simulink model "Deploy_Simulink_R2015b"  (R2015b)
settings: Solver=ode1  StartTime=0.0  StopTime=inf  FixedStep=0.004  RelTol=1e-3
values from neighbouring files (symbols this model uses):
  elev_0 = -27.5*pi/180    (= -0.479965544298)    [setup_lab_heli_3d.m]
  K_AMP = 3    [setup_lab_heli_3d.m]
  K_EC_E = - 2 * pi / ( 4 * 1024 )    (= -0.00153398078789)    [setup_heli_3d_configuration.m]
  K_EC_P = 2 * pi / ( 4 * 1024 )    (= 0.00153398078789)    [setup_heli_3d_configuration.m]
  K_EC_T = 2 * pi / ( 8 * 1024 )    (= 0.000766990393943)    [setup_heli_3d_configuration.m]
  lambdaSplit = reshape(lambda, lambdaDim,  sizeSeg,DoP)    [Simulink_Setup.m]
  LAMBDASplit = reshape(LAMBDA, xDim, xDim, sizeSeg,DoP)    [Simulink_Setup.m]
  pSplit = reshape(par,    pDim,       sizeSeg,DoP)    [Simulink_Setup.m]
  uSplit = reshape(u,      uDim,       sizeSeg,DoP)    [Simulink_Setup.m]
  VMAX_AMP = 24    [setup_lab_heli_3d.m]
  VMAX_DAC = 10    [setup_lab_heli_3d.m]
  wcf = 2 * pi * 4    (= 25.1327412287)    [setup_lab_heli_3d.m]
  xSplit = reshape(x,      xDim,       sizeSeg,DoP)    [Simulink_Setup.m]
  zetaf = 0.9    [setup_lab_heli_3d.m]
undefined symbols (not defined in the file or in its folder): HIL, qc_get_step_size
libraries: quarc_library x4
settings Model: SimulationMode=external  Creator=Deng  LastModifiedBy=deng
settings SolverCC: PositivePriorityOrder=on
settings DataIOCC: LimitDataPoints=off
settings OptimizationCC: SimCompilerOptimization=on
settings DebuggingCC: AllowSymbolicDim=on
settings HardwareCC: ProdBitPerPointer=32  ProdLargestAtomicFloat=None  ProdWordSize=32  ProdHWDeviceType=Custom Processor->Custom
settings ModelReferenceCC: PropagateSignalLabelsOutOfModel=on
settings SFSimCC: SimCustomHeaderCode="#include \"NMPC_Iter.h\""  SimUserSources=NMPC_Iter.c OCP_F_Fu_Fx.c  SimUserLibraries=NMPC_Iter.lib
settings SFSimCC: SimUserIncludeDirs=|
  | .\codegen\lib\NMPC_Iter
  | .\codegen\lib\OCP_F_Fu_Fx
settings RTWCC: SystemTargetFile=quarc_win64.tlc  TemplateMakefile=quarc_default_tmf  Description=QUARC Win64 Target  GenerateReport=on  RTWUseSimCustomCode=on  CustomHeaderCode="#include \"NMPC_Iter.h\""  CustomSource=NMPC_Iter.c OCP_F_Fu_Fx.c  CustomLibrary=NMPC_Iter.lib  BuildConfiguration=Faster Runs  LaunchReport=on
settings RTWCC: CustomInclude=|
  | .\codegen\lib\NMPC_Iter
  | .\codegen\lib\OCP_F_Fu_Fx
settings STFCustomTargetCC: GeneratePreprocessorConditionals=Use local settings  CPPClassGenCompliant=off
settings GRTTargetCC: ParMdlRefBuildCompliant=off  CompOptLevelCompliant=off  CombineOutputUpdateFcns=off  MatFileLogging=off  CPPClassGenCompliant=off  GRTInterface=on  UseToolchainInfoCompliant=off  ExtMode=on  ExtModeMexFile=quarc_comm

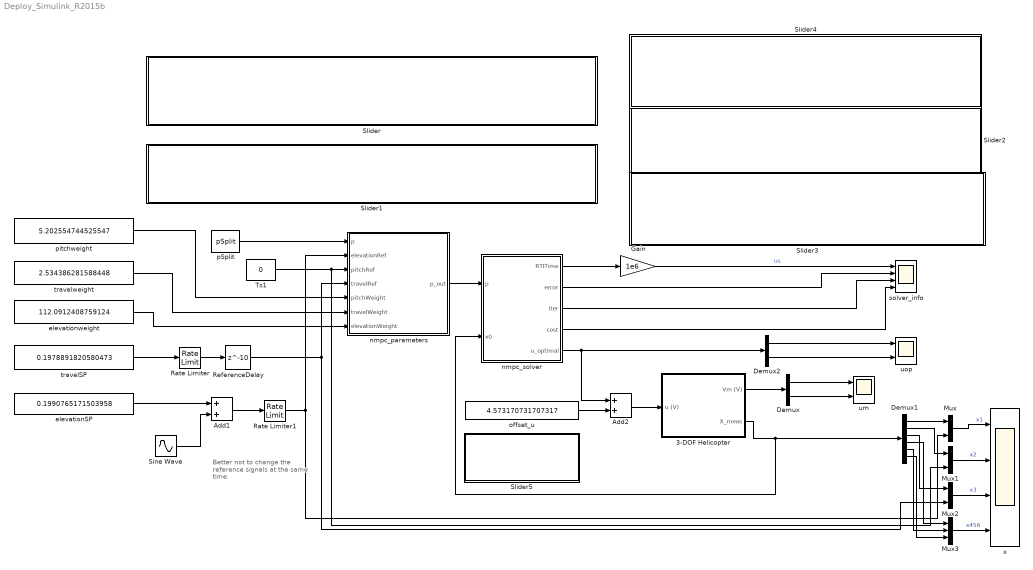
== system Deploy_Simulink_R2015b ==
  note: Better not to change the reference signals at the same time.
  3-DOF Helicopter : Subsystem
  Add1 : Sum
  Add2 : Sum
  Demux : Demux  Outputs=2
  Demux1 : Demux  Outputs=6
  Demux2 : Demux  Outputs=2
  Gain : Gain  Gain=1e6
  Mux : Mux  Inputs=2
  Mux1 : Mux  Inputs=2
  Mux2 : Mux  Inputs=2
  Mux3 : Mux  Inputs=3
  Rate Limiter : RateLimiter  RisingSlewLimit=2  FallingSlewLimit=-2  SampleTimeMode=inherited
  Rate Limiter1 : RateLimiter  RisingSlewLimit=50  FallingSlewLimit=-50  SampleTimeMode=inherited
  ReferenceDelay : Delay  DelayLength=10  InitialCondition=0
  Sine Wave : Sin  Amplitude=0  Frequency=0.5  SampleTime=0
  Slider : Subsystem  DialogController=hmiCreateDDGDialog  IsWebBlock=on  mask(MWDashboardBlock){webBlockId=958bdc94-fbbd-4d66-a7c2-c7b380b51c1f, webBlockType=slider, ShowInLibBrowser=on, ShowInitialText=on, HMISrcModelName=Simulink_C_Deploy_R2015b}
      mask prompts: webBlockId "WebBlock Id"; webBlockType "WebBlock Type"; HMISrcModelName "Source Model"
      mask Help: helpview([docroot '/mapfiles/simulink.map'], 'hmi_slider')
      mask Display:
      | if strcmp(get_param(bdroot(gcb),'BlockDiagramType'), 'library')
      |     image([(matlabroot) '/toolbox/simulink/hmi/icons/Slider.png']);
      | end
  Slider1 : Subsystem  DialogController=hmiCreateDDGDialog  IsWebBlock=on  mask(MWDashboardBlock){webBlockId=d0239637-77bd-428c-ab30-bd13650fc7b6, webBlockType=slider, ShowInLibBrowser=on, ShowInitialText=on, HMISrcModelName=Simulink_C_Deploy_R2015b}
      mask prompts: webBlockId "WebBlock Id"; webBlockType "WebBlock Type"; HMISrcModelName "Source Model"
      mask Help: helpview([docroot '/mapfiles/simulink.map'], 'hmi_slider')
      mask Display:
      | if strcmp(get_param(bdroot(gcb),'BlockDiagramType'), 'library')
      |     image([(matlabroot) '/toolbox/simulink/hmi/icons/Slider.png']);
      | end
  Slider2 : Subsystem  DialogController=hmiCreateDDGDialog  IsWebBlock=on  mask(MWDashboardBlock){webBlockId=9382aac3-409f-4dab-a4f9-baf18b7ce907, webBlockType=slider, ShowInLibBrowser=on, ShowInitialText=on, HMISrcModelName=Simulink_C_Deploy_R2015b}
      mask prompts: webBlockId "WebBlock Id"; webBlockType "WebBlock Type"; HMISrcModelName "Source Model"
      mask Help: helpview([docroot '/mapfiles/simulink.map'], 'hmi_slider')
      mask Display:
      | if strcmp(get_param(bdroot(gcb),'BlockDiagramType'), 'library')
      |     image([(matlabroot) '/toolbox/simulink/hmi/icons/Slider.png']);
      | end
  Slider3 : Subsystem  DialogController=hmiCreateDDGDialog  IsWebBlock=on  mask(MWDashboardBlock){webBlockId=d7a49558-d97e-4fdd-ae2b-0498040a2635, webBlockType=slider, ShowInLibBrowser=on, ShowInitialText=on, HMISrcModelName=Simulink_C_Deploy_R2015b}
      mask prompts: webBlockId "WebBlock Id"; webBlockType "WebBlock Type"; HMISrcModelName "Source Model"
      mask Help: helpview([docroot '/mapfiles/simulink.map'], 'hmi_slider')
      mask Display:
      | if strcmp(get_param(bdroot(gcb),'BlockDiagramType'), 'library')
      |     image([(matlabroot) '/toolbox/simulink/hmi/icons/Slider.png']);
      | end
  Slider4 : Subsystem  DialogController=hmiCreateDDGDialog  IsWebBlock=on  mask(MWDashboardBlock){webBlockId=5022bdd5-4ec7-4769-8c29-2847bff93344, webBlockType=slider, ShowInLibBrowser=on, ShowInitialText=on, HMISrcModelName=Simulink_C_Deploy_R2015b}
      mask prompts: webBlockId "WebBlock Id"; webBlockType "WebBlock Type"; HMISrcModelName "Source Model"
      mask Help: helpview([docroot '/mapfiles/simulink.map'], 'hmi_slider')
      mask Display:
      | if strcmp(get_param(bdroot(gcb),'BlockDiagramType'), 'library')
      |     image([(matlabroot) '/toolbox/simulink/hmi/icons/Slider.png']);
      | end
  Slider5 : Subsystem  DialogController=hmiCreateDDGDialog  IsWebBlock=on  mask(MWDashboardBlock){webBlockId=dba8a8ef-8cf2-4f6b-b7e7-21e88edd4f6f, webBlockType=slider, ShowInLibBrowser=on, ShowInitialText=on, HMISrcModelName=Simulink_C_Deploy_R2015b}
      mask prompts: webBlockId "WebBlock Id"; webBlockType "WebBlock Type"; HMISrcModelName "Source Model"
      mask Help: helpview([docroot '/mapfiles/simulink.map'], 'hmi_slider')
      mask Display:
      | if strcmp(get_param(bdroot(gcb),'BlockDiagramType'), 'library')
      |     image([(matlabroot) '/toolbox/simulink/hmi/icons/Slider.png']);
      | end
  Ts1 : Constant  Value=0
  elevationSP : Constant  Value=0.1990765171503958
  elevationweight : Constant  Value=112.0912408759124
  nmpc_parameters : MATLAB Function  TreatAsAtomicUnit=on
  nmpc_solver : Subsystem
  offset_u : Constant  Value=4.573170731707317
  pSplit : Constant  Value=pSplit
  pitchweight : Constant  Value=5.202554744525547
  solver_info : Scope  NumInputPorts=4
  travelSP : Constant  Value=0.1978891820580473
  travelweight : Constant  Value=2.534386281588448
  um : Scope  NumInputPorts=2
  uop : Scope  NumInputPorts=2
  x : Scope  NumInputPorts=4
  wires:
  pSplit/1 -> nmpc_parameters/1(p)
  nmpc_parameters/1(p_out) -> nmpc_solver/1(p)
  nmpc_solver/2(error) -> solver_info/2
  nmpc_solver/1(RTITime) -> Gain/1
  nmpc_solver/4(cost) -> solver_info/4
  nmpc_solver/3(iter) -> solver_info/3
  Gain/1 -> solver_info/1  "us"
  Ts1/1 -> nmpc_parameters/3(pitchRef), Mux1/2
  Demux/1 -> um/1
  Demux/2 -> um/2
  3-DOF Helicopter/2(X_meas) -> nmpc_solver/2(x0), Demux1/1
  Rate Limiter/1 -> ReferenceDelay/1
  Rate Limiter1/1 -> Mux/2, nmpc_parameters/2(elevationRef)
  Demux1/1 -> Mux/1
  Mux/1 -> x/1  "x1"
  Demux1/2 -> Mux1/1
  Mux1/1 -> x/2  "x2"
  Mux2/1 -> x/3  "x3"
  Demux1/3 -> Mux2/1
  Demux1/4 -> Mux3/1
  Demux1/5 -> Mux3/2
  Demux1/6 -> Mux3/3
  Mux3/1 -> x/4  "x456"
  ReferenceDelay/1 -> nmpc_parameters/4(travelRef), Mux2/2
  elevationSP/1 -> Add1/1
  Add1/1 -> Rate Limiter1/1
  Sine Wave/1 -> Add1/2
  travelSP/1 -> Rate Limiter/1
  Add2/1 -> 3-DOF Helicopter/1(u (V))
  3-DOF Helicopter/1(Vm (V)) -> Demux/1
  Demux2/1 -> uop/1
  Demux2/2 -> uop/2
  pitchweight/1 -> nmpc_parameters/5(pitchWeight)
  travelweight/1 -> nmpc_parameters/6(travelWeight)
  elevationweight/1 -> nmpc_parameters/7(elevationWeight)
  nmpc_solver/5(u_optimal) -> Add2/1, Demux2/1
  offset_u/1 -> Add2/2

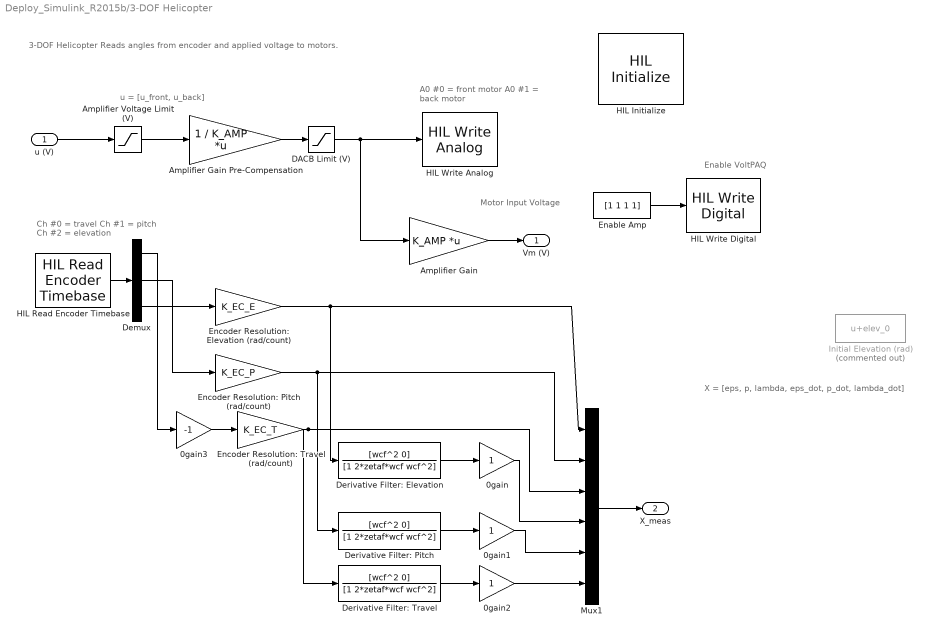
== system Deploy_Simulink_R2015b/3-DOF Helicopter ==
  note: A0 #0 = front motor
      | A0 #1 = back motor
  note: u = [u_front, u_back]
  note: Motor Input Voltage
  note: 3-DOF Helicopter
      | Reads angles from encoder and applied voltage to motors.
  note: Ch #0 = travel
      | Ch #1 = pitch
      | Ch #2 = elevation
  note: X = [eps, p, lambda, eps_dot, p_dot, lambda_dot]
  note: Enable VoltPAQ
  u (V) : Inport
  0gain : Gain
  0gain1 : Gain
  0gain2 : Gain
  0gain3 : Gain  Gain=-1
  Amplifier Gain : Gain  Gain=K_AMP  Multiplication=Matrix(K*u)  SaturateOnIntegerOverflow=on  OutDataTypeStr=Inherit: Same as input  ParamDataTypeStr=Inherit: Same as input
  Amplifier Gain Pre-Compensation : Gain  Gain=1 / K_AMP  Multiplication=Matrix(K*u)  SaturateOnIntegerOverflow=on  OutDataTypeStr=Inherit: Same as input  ParamDataTypeStr=Inherit: Same as input
  Amplifier Voltage Limit (V) : Saturate  UpperLimit=VMAX_AMP  LowerLimit=0
  DACB Limit (V) : Saturate  UpperLimit=VMAX_DAC  LowerLimit=-VMAX_DAC
  Demux : Demux  Outputs=3
  Derivative Filter: Elevation : TransferFcn  Numerator=[wcf^2 0]  Denominator=[1 2*zetaf*wcf wcf^2]
  Derivative Filter: Pitch : TransferFcn  Numerator=[wcf^2 0]  Denominator=[1 2*zetaf*wcf wcf^2]
  Derivative Filter: Travel : TransferFcn  Numerator=[wcf^2 0]  Denominator=[1 2*zetaf*wcf wcf^2]
  Enable Amp : Constant  Value=[1 1 1 1]
  Encoder Resolution: Elevation (rad/count) : Gain  Gain=K_EC_E
  Encoder Resolution: Pitch (rad/count) : Gain  Gain=K_EC_P
  Encoder Resolution: Travel (rad/count) : Gain  Gain=K_EC_T
  HIL Initialize : quarc_library/Data Acquisition/Generic/Configuration/HIL Initialize  object_name=HIL-1  board_type=q8_usb  board_number=0  board_options=update_rate=normal  exclusive=off  active=on  hardware_clocks=[0:2]  clock_modes=[]  initial_clock_frequencies=[]  set_clock_params_at_start=off  set_clock_params_at_switch_in=off  set_clock_frequencies_at_start=off  set_clock_frequencies_at_switch_in=off  analog_input_channels=[0:7]  analog_input_configurations=[]  analog_input_maximums=10  analog_input_minimums=-10  set_analog_input_params_at_start=on  set_analog_input_params_at_switch_in=off  analog_output_channels=[0:7]  analog_output_maximums=10  analog_output_minimums=-10  initial_analog_outputs=[0]  final_analog_outputs=[0]  watchdog_analog_outputs=0  set_analog_output_params_at_start=on  set_analog_output_params_at_switch_in=off  set_analog_outputs_at_start=on  set_analog_outputs_at_switch_in=off  set_analog_outputs_at_terminate=on  set_analog_outputs_at_switch_out=off  set_analog_outputs_on_watchdog=off  digital_input_channels=[4:7]  digital_output_channels=[0:3]  digital_output_configuration=[]  initial_digital_outputs=[0]  final_digital_outputs=[0]  watchdog_digital_outputs=[0]  set_digital_output_params_at_start=off  set_digital_output_params_at_switch_in=off  set_digital_outputs_at_start=on  set_digital_outputs_at_switch_in=off  set_digital_outputs_at_terminate=on  set_digital_outputs_at_switch_out=off  set_digital_outputs_on_watchdog=off  encoder_channels=[0:7]  quadrature=[4]  encoder_filter_frequency=[]  initial_encoder_counts=[0]  set_encoder_params_at_start=on  set_encoder_params_at_switch_in=off  set_encoder_counts_at_start=on  set_encoder_counts_at_switch_in=off  pwm_channels=[0:7]  pwm_modes=0  pwm_frequency=99.532799999999995e6/4095  pwm_configuration=[0]  pwm_alignment=[0]  pwm_polarity=[1]  pwm_leading_deadband=[0]  pwm_trailing_deadband=[0]  initial_pwm_outputs=[0]  final_pwm_outputs=[0]  watchdog_pwm_outputs=[0]  set_pwm_params_at_start=on  set_pwm_params_at_switch_in=off  set_pwm_outputs_at_start=on  set_pwm_outputs_at_switch_in=off  set_pwm_outputs_at_terminate=on  set_pwm_outputs_at_switch_out=off  set_pwm_outputs_on_watchdog=off  other_output_channels=[]  initial_other_outputs=[]  final_other_outputs=[]  watchdog_other_outputs=[]  set_other_outputs_at_start=off  set_other_outputs_at_switch_in=off  set_other_outputs_at_terminate=off  set_other_outputs_at_switch_out=off  set_other_outputs_on_watchdog=off
  HIL Read Encoder Timebase : quarc_library/Data Acquisition/Generic/Timebases/HIL Read Encoder Timebase  object_name=HIL-1  clock=0  channels=[0:2]  samples_in_buffer=max(ceil(1/qc_get_step_size), 1)  active=on  vector_output=on  data_type_mode=Inherit via back propagation  data_type=double
  HIL Write Analog : quarc_library/Data Acquisition/Generic/Immediate I//O/HIL Write Analog  object_name=HIL-1  channels=[0,1]  sample_time=-1  active=off  vector_input=on
  HIL Write Digital : quarc_library/Data Acquisition/Generic/Immediate I//O/HIL Write Digital  object_name=HIL-1  channels=[0:3]  sample_time=-1  active=off  vector_input=on
  Initial Elevation (rad) : Bias  Commented=on  Bias=elev_0
  Mux1 : Mux  Inputs=6
  Vm (V) : Outport
  X_meas : Outport  Port=2
  wires:
  HIL Read Encoder Timebase/1 -> Demux/1
  Mux1/1 -> X_meas/1
  Amplifier Gain Pre-Compensation/1 -> DACB Limit (V)/1
  Amplifier Voltage Limit (V)/1 -> Amplifier Gain Pre-Compensation/1
  Amplifier Gain/1 -> Vm (V)/1
  u (V)/1 -> Amplifier Voltage Limit (V)/1
  DACB Limit (V)/1 -> Amplifier Gain/1, HIL Write Analog/1
  Demux/3 -> Encoder Resolution: Elevation (rad/count)/1
  Demux/1 -> 0gain3/1
  Demux/2 -> Encoder Resolution: Pitch (rad/count)/1
  Encoder Resolution: Pitch (rad/count)/1 -> Mux1/2, Derivative Filter: Pitch/1
  Encoder Resolution: Elevation (rad/count)/1 -> Derivative Filter: Elevation/1, Mux1/1
  Enable Amp/1 -> HIL Write Digital/1
  Derivative Filter: Travel/1 -> 0gain2/1
  Derivative Filter: Pitch/1 -> 0gain1/1
  Derivative Filter: Elevation/1 -> 0gain/1
  0gain/1 -> Mux1/4
  0gain1/1 -> Mux1/5
  0gain2/1 -> Mux1/6
  Encoder Resolution: Travel (rad/count)/1 -> Derivative Filter: Travel/1, Mux1/3
  0gain3/1 -> Encoder Resolution: Travel (rad/count)/1

== system Deploy_Simulink_R2015b/Slider ==

== system Deploy_Simulink_R2015b/Slider1 ==

== system Deploy_Simulink_R2015b/Slider2 ==

== system Deploy_Simulink_R2015b/Slider3 ==

== system Deploy_Simulink_R2015b/Slider4 ==

== system Deploy_Simulink_R2015b/Slider5 ==

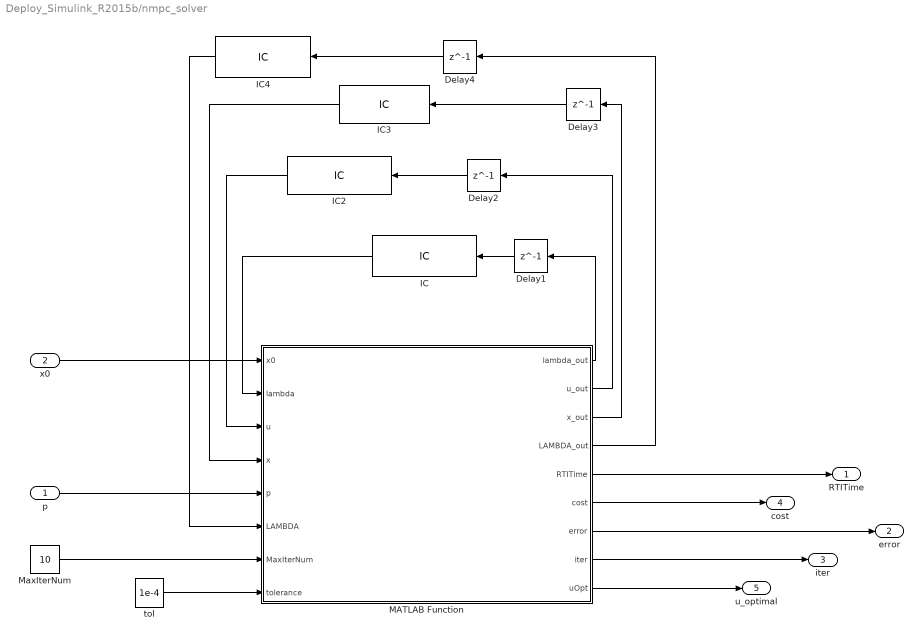
== system Deploy_Simulink_R2015b/nmpc_solver ==
  p : Inport
  x0 : Inport  Port=2
  Delay{1..4} (4 alike) : Delay  DelayLength=1  InitialCondition=0
  IC : InitialCondition  Value=lambdaSplit
  IC2 : InitialCondition  Value=uSplit
  IC3 : InitialCondition  Value=xSplit
  IC4 : InitialCondition  Value=LAMBDASplit
  MATLAB Function : MATLAB Function  TreatAsAtomicUnit=on
  MaxIterNum : Constant  Value=10
  tol : Constant  Value=1e-4
  RTITime : Outport
  error : Outport  Port=2
  iter : Outport  Port=3
  cost : Outport  Port=4
  u_optimal : Outport  Port=5
  wires:
  Delay2/1 -> IC2/1
  Delay1/1 -> IC/1
  Delay4/1 -> IC4/1
  Delay3/1 -> IC3/1
  x0/1 -> MATLAB Function/1(x0)
  IC/1 -> MATLAB Function/2(lambda)
  IC2/1 -> MATLAB Function/3(u)
  IC3/1 -> MATLAB Function/4(x)
  IC4/1 -> MATLAB Function/6(LAMBDA)
  p/1 -> MATLAB Function/5(p)
  MaxIterNum/1 -> MATLAB Function/7(MaxIterNum)
  tol/1 -> MATLAB Function/8(tolerance)
  MATLAB Function/1(lambda_out) -> Delay1/1
  MATLAB Function/2(u_out) -> Delay2/1
  MATLAB Function/4(LAMBDA_out) -> Delay4/1
  MATLAB Function/5(RTITime) -> RTITime/1
  MATLAB Function/6(cost) -> cost/1
  MATLAB Function/7(error) -> error/1
  MATLAB Function/9(uOpt) -> u_optimal/1
  MATLAB Function/3(x_out) -> Delay3/1
  MATLAB Function/8(iter) -> iter/1

== matlab function Deploy_Simulink_R2015b/nmpc_solver/MATLAB Function ==
  data: lambda_out output; u_out output; x_out output; LAMBDA_out output; RTITime output; cost output; error output; iter output; uOpt output; x0 input; lambda input; u input; x input; p input; LAMBDA input; MaxIterNum input; tolerance input
function [lambda_out,u_out, x_out, LAMBDA_out, RTITime, cost, error, iter, uOpt]= ...
                        MATLAB_Function(...
                        x0,...
                        lambda,...
                        u,...
                        x, p, LAMBDA, MaxIterNum, tolerance)
%#codegen
cost = 0;
error = 0;
timeElapsed = 0;
RTITime = 0;

coder.ceval('NMPC_Iter_initialize');
for iter=1:MaxIterNum
    % Executing in generated code, call C function 
    coder.ceval('NMPC_Iter',...
                  x0,...
                  coder.ref(lambda),...
                  coder.ref(u),...
                  coder.ref(x),...
                  coder.ref(p),...
                  coder.ref(LAMBDA),...
                  coder.wref(cost),...
                  coder.wref(error),...
                  coder.wref(timeElapsed));
    RTITime = RTITime + timeElapsed;
    if error<tolerance
        break;
    end
end
lambda_out =  lambda;
u_out =  u;
x_out =  x;
LAMBDA_out=  LAMBDA;
uOpt = u(1:2);

== matlab function Deploy_Simulink_R2015b/nmpc_parameters ==
  data: p input; elevationRef input; pitchRef input; travelRef input; p_out output; pitchWeight input; travelWeight input; elevationWeight input
function p_out = nmpc_parameters(p,elevationRef,pitchRef, travelRef,pitchWeight,travelWeight,elevationWeight)
%#codegen
p_out = p;
p_out(9,:,:) = elevationRef;
p_out(10,:,:) = pitchRef;
p_out(11,:,:) = travelRef;
p_out(1,:,:) = elevationWeight;
p_out(2,:,:) = pitchWeight;
p_out(3,:,:) = travelWeight;
